simulink model "JingChuJointR"  (R2025b)
settings: Solver=VariableStepAuto  StartTime=0.0  StopTime=10.0  RelTol=1e-3
undefined symbols (not defined in the file or in its folder): X, Y, Z
libraries: sm_lib x486, nesl_utility x6
(part 9 of 9)

== system JingChuJointR/waist_roll1 ==
  Inertia : sm_lib/Body Elements/Inertia  InertiaType=Custom  Mass=1.815  MassUnits=kg  CenterOfMass=[0, 0, 0]  CenterOfMassUnits=m  MomentsOfInertia=[0.002180655, 0.00238951, 0.002296057]  MomentsOfInertiaUnits=kg*m^2  ProductsOfInertia=[-3.6e-08, -8.354199999999999e-05, -8e-09]  ProductsOfInertiaUnits=kg*m^2  GraphicType=None  MarkerShape=Inertia  MarkerSize=20  GraphicVisPropType=SimpleVisualProperties  GraphicDiffuseColor=[0.5 0.5 0.5]  GraphicOpacity=1  GraphicSpecularColor=[0.5 0.5 0.5 1.0]  GraphicAmbientColor=[0.15 0.15 0.15 1.0]  GraphicEmissiveColor=[0.0 0.0 0.0 1.0]  GraphicShininess=75
  InertiaOriginTransform : sm_lib/Frames and Transforms/Rigid Transform  RotationMethod=RotationSequence  FollAlignAxisA=+X  BaseAlignAxisA=+Y  FollAlignAxisB=+Y  BaseAlignAxisB=+Z  RotationStandardAxis=+Z  RotationAngle=0  RotationAngleUnits=deg  RotationArbitraryAxis=[0 0 1]  RotationSequenceAxes=BaseAxes  RotationSequence=XYZ  RotationSequenceAngles=[0, 0, 0]  RotationSequenceAnglesUnits=rad  RotationMatrix=[1 0 0;0 1 0;0 0 1]  Quaternion=[1 0 0 0]  TranslationMethod=Cartesian  TranslationCartesianOffset=[-0.004186, 0, -0.006951]  TranslationCartesianOffsetUnits=m  TranslationStandardAxis=+Z  TranslationStandardOffset=0  TranslationStandardOffsetUnits=m  TranslationROffset=0  TranslationROffsetUnits=m  TranslationThetaOffset=0  TranslationThetaOffsetUnits=deg  TranslationZOffset=0  TranslationZOffsetUnits=m
  ReferenceFrame : sm_lib/Frames and Transforms/Reference Frame
  Visual : sm_lib/Body Elements/File Solid  ExtGeomFileName=./meshes/waist_roll.STL  UnitType=Custom  ExtGeomFileUnits=m  StepReaderType=HEX  ExportConvexHullGeometry=off  InertiaType=Custom  BasedOnType=DensityFromFile  Density=1000  DensityUnits=kg/m^3  Mass=0  MassUnits=kg  CenterOfMass=[0, 0, 0]  CenterOfMassUnits=m  MomentsOfInertia=[0, 0, 0]  MomentsOfInertiaUnits=kg*m^2  ProductsOfInertia=[0, 0, 0]  ProductsOfInertiaUnits=kg*m^2  GraphicType=FromGeometry  MarkerShape=Sphere  MarkerSize=10  GraphicVisPropType=SimpleVisualProperties  GraphicDiffuseColor=[1, 1, 1]  GraphicOpacity=1  GraphicSpecularColor=[0.5 0.5 0.5 1.0]  GraphicAmbientColor=[0.15 0.15 0.15 1.0]  GraphicEmissiveColor=[0.0 0.0 0.0 1.0]  GraphicShininess=75  DoExposeReferenceFrame=on  SerializedFrames=<Frames/>
  VisualOriginTransform : sm_lib/Frames and Transforms/Rigid Transform  RotationMethod=RotationSequence  FollAlignAxisA=+X  BaseAlignAxisA=+Y  FollAlignAxisB=+Y  BaseAlignAxisB=+Z  RotationStandardAxis=+Z  RotationAngle=0  RotationAngleUnits=deg  RotationArbitraryAxis=[0 0 1]  RotationSequenceAxes=BaseAxes  RotationSequence=XYZ  RotationSequenceAngles=[0, 0, 0]  RotationSequenceAnglesUnits=rad  RotationMatrix=[1 0 0;0 1 0;0 0 1]  Quaternion=[1 0 0 0]  TranslationMethod=Cartesian  TranslationCartesianOffset=[0, 0, 0]  TranslationCartesianOffsetUnits=m  TranslationStandardAxis=+Z  TranslationStandardOffset=0  TranslationStandardOffsetUnits=m  TranslationROffset=0  TranslationROffsetUnits=m  TranslationThetaOffset=0  TranslationThetaOffsetUnits=deg  TranslationZOffset=0  TranslationZOffsetUnits=m
  waist_roll_AxisInvTransform : sm_lib/Frames and Transforms/Rigid Transform  RotationMethod=ArbitraryAxis  FollAlignAxisA=+X  BaseAlignAxisA=+Y  FollAlignAxisB=+Y  BaseAlignAxisB=+Z  RotationStandardAxis=+Z  RotationAngle=1.570796326794897  RotationAngleUnits=rad  RotationArbitraryAxis=[-0, 1, 0]  RotationSequenceAxes=FollowerAxes  RotationSequence=XYX  RotationSequenceAngles=[0 0 0]  RotationSequenceAnglesUnits=deg  RotationMatrix=[1 0 0;0 1 0;0 0 1]  Quaternion=[1 0 0 0]  TranslationMethod=Cartesian  TranslationCartesianOffset=[0, 0, 0]  TranslationCartesianOffsetUnits=m  TranslationStandardAxis=+Z  TranslationStandardOffset=0  TranslationStandardOffsetUnits=m  TranslationROffset=0  TranslationROffsetUnits=m  TranslationThetaOffset=0  TranslationThetaOffsetUnits=deg  TranslationZOffset=0  TranslationZOffsetUnits=m
  waist_yaw_AxisTransform : sm_lib/Frames and Transforms/Rigid Transform  RotationMethod=ArbitraryAxis  FollAlignAxisA=+X  BaseAlignAxisA=+Y  FollAlignAxisB=+Y  BaseAlignAxisB=+Z  RotationStandardAxis=+Z  RotationAngle=0  RotationAngleUnits=rad  RotationArbitraryAxis=[1, 0, 0]  RotationSequenceAxes=FollowerAxes  RotationSequence=XYX  RotationSequenceAngles=[0 0 0]  RotationSequenceAnglesUnits=deg  RotationMatrix=[1 0 0;0 1 0;0 0 1]  Quaternion=[1 0 0 0]  TranslationMethod=Cartesian  TranslationCartesianOffset=[0, 0, 0]  TranslationCartesianOffsetUnits=m  TranslationStandardAxis=+Z  TranslationStandardOffset=0  TranslationStandardOffsetUnits=m  TranslationROffset=0  TranslationROffsetUnits=m  TranslationThetaOffset=0  TranslationThetaOffsetUnits=deg  TranslationZOffset=0  TranslationZOffsetUnits=m
  waist_yaw_OriginTransform : sm_lib/Frames and Transforms/Rigid Transform  RotationMethod=RotationSequence  FollAlignAxisA=+X  BaseAlignAxisA=+Y  FollAlignAxisB=+Y  BaseAlignAxisB=+Z  RotationStandardAxis=+Z  RotationAngle=0  RotationAngleUnits=deg  RotationArbitraryAxis=[0 0 1]  RotationSequenceAxes=BaseAxes  RotationSequence=XYZ  RotationSequenceAngles=[0, 0, 0]  RotationSequenceAnglesUnits=rad  RotationMatrix=[1 0 0;0 1 0;0 0 1]  Quaternion=[1 0 0 0]  TranslationMethod=Cartesian  TranslationCartesianOffset=[0, 0, 0]  TranslationCartesianOffsetUnits=m  TranslationStandardAxis=+Z  TranslationStandardOffset=0  TranslationStandardOffsetUnits=m  TranslationROffset=0  TranslationROffsetUnits=m  TranslationThetaOffset=0  TranslationThetaOffsetUnits=deg  TranslationZOffset=0  TranslationZOffsetUnits=m
  F : PMIOPort  Side=Left
  F1 : PMIOPort  Port=2  Side=Right
  connections:
  Inertia/RConn1 -- InertiaOriginTransform/RConn1
  ReferenceFrame/RConn1 -- InertiaOriginTransform/LConn1 -- VisualOriginTransform/LConn1 -- waist_roll_AxisInvTransform/LConn1 -- waist_yaw_OriginTransform/LConn1
  Visual/RConn1 -- VisualOriginTransform/RConn1
  waist_roll_AxisInvTransform/RConn1 -- F/RConn1
  waist_yaw_AxisTransform/RConn1 -- F1/RConn1
  waist_yaw_AxisTransform/LConn1 -- waist_yaw_OriginTransform/RConn1

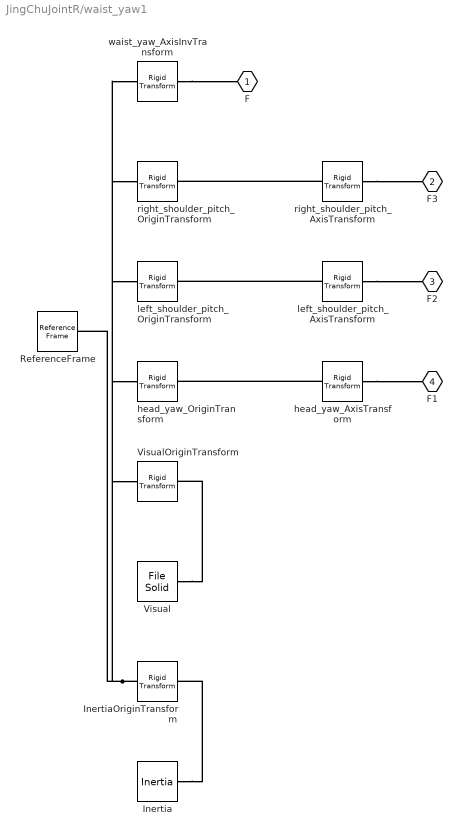
== system JingChuJointR/waist_yaw1 ==
  Inertia : sm_lib/Body Elements/Inertia  InertiaType=Custom  Mass=16.823  MassUnits=kg  CenterOfMass=[0, 0, 0]  CenterOfMassUnits=m  MomentsOfInertia=[0.256789087, 0.21861739, 0.122453074]  MomentsOfInertiaUnits=kg*m^2  ProductsOfInertia=[-0.000143525, 0.007865723, -9.021000000000001e-06]  ProductsOfInertiaUnits=kg*m^2  GraphicType=None  MarkerShape=Inertia  MarkerSize=20  GraphicVisPropType=SimpleVisualProperties  GraphicDiffuseColor=[0.5 0.5 0.5]  GraphicOpacity=1  GraphicSpecularColor=[0.5 0.5 0.5 1.0]  GraphicAmbientColor=[0.15 0.15 0.15 1.0]  GraphicEmissiveColor=[0.0 0.0 0.0 1.0]  GraphicShininess=75
  InertiaOriginTransform : sm_lib/Frames and Transforms/Rigid Transform  RotationMethod=RotationSequence  FollAlignAxisA=+X  BaseAlignAxisA=+Y  FollAlignAxisB=+Y  BaseAlignAxisB=+Z  RotationStandardAxis=+Z  RotationAngle=0  RotationAngleUnits=deg  RotationArbitraryAxis=[0 0 1]  RotationSequenceAxes=BaseAxes  RotationSequence=XYZ  RotationSequenceAngles=[0, 0, 0]  RotationSequenceAnglesUnits=rad  RotationMatrix=[1 0 0;0 1 0;0 0 1]  Quaternion=[1 0 0 0]  TranslationMethod=Cartesian  TranslationCartesianOffset=[-0.04269, 3e-05, 0.24319]  TranslationCartesianOffsetUnits=m  TranslationStandardAxis=+Z  TranslationStandardOffset=0  TranslationStandardOffsetUnits=m  TranslationROffset=0  TranslationROffsetUnits=m  TranslationThetaOffset=0  TranslationThetaOffsetUnits=deg  TranslationZOffset=0  TranslationZOffsetUnits=m
  ReferenceFrame : sm_lib/Frames and Transforms/Reference Frame
  Visual : sm_lib/Body Elements/File Solid  ExtGeomFileName=./meshes/waist_yaw.STL  UnitType=Custom  ExtGeomFileUnits=m  StepReaderType=HEX  ExportConvexHullGeometry=off  InertiaType=Custom  BasedOnType=DensityFromFile  Density=1000  DensityUnits=kg/m^3  Mass=0  MassUnits=kg  CenterOfMass=[0, 0, 0]  CenterOfMassUnits=m  MomentsOfInertia=[0, 0, 0]  MomentsOfInertiaUnits=kg*m^2  ProductsOfInertia=[0, 0, 0]  ProductsOfInertiaUnits=kg*m^2  GraphicType=FromGeometry  MarkerShape=Sphere  MarkerSize=10  GraphicVisPropType=SimpleVisualProperties  GraphicDiffuseColor=[1, 1, 1]  GraphicOpacity=1  GraphicSpecularColor=[0.5 0.5 0.5 1.0]  GraphicAmbientColor=[0.15 0.15 0.15 1.0]  GraphicEmissiveColor=[0.0 0.0 0.0 1.0]  GraphicShininess=75  DoExposeReferenceFrame=on  SerializedFrames=<Frames/>
  VisualOriginTransform : sm_lib/Frames and Transforms/Rigid Transform  RotationMethod=RotationSequence  FollAlignAxisA=+X  BaseAlignAxisA=+Y  FollAlignAxisB=+Y  BaseAlignAxisB=+Z  RotationStandardAxis=+Z  RotationAngle=0  RotationAngleUnits=deg  RotationArbitraryAxis=[0 0 1]  RotationSequenceAxes=BaseAxes  RotationSequence=XYZ  RotationSequenceAngles=[0, 0, 0]  RotationSequenceAnglesUnits=rad  RotationMatrix=[1 0 0;0 1 0;0 0 1]  Quaternion=[1 0 0 0]  TranslationMethod=Cartesian  TranslationCartesianOffset=[0, 0, 0]  TranslationCartesianOffsetUnits=m  TranslationStandardAxis=+Z  TranslationStandardOffset=0  TranslationStandardOffsetUnits=m  TranslationROffset=0  TranslationROffsetUnits=m  TranslationThetaOffset=0  TranslationThetaOffsetUnits=deg  TranslationZOffset=0  TranslationZOffsetUnits=m
  head_yaw_AxisTransform : sm_lib/Frames and Transforms/Rigid Transform  RotationMethod=ArbitraryAxis  FollAlignAxisA=+X  BaseAlignAxisA=+Y  FollAlignAxisB=+Y  BaseAlignAxisB=+Z  RotationStandardAxis=+Z  RotationAngle=3.141592653589793  RotationAngleUnits=rad  RotationArbitraryAxis=[1, 0, 0]  RotationSequenceAxes=FollowerAxes  RotationSequence=XYX  RotationSequenceAngles=[0 0 0]  RotationSequenceAnglesUnits=deg  RotationMatrix=[1 0 0;0 1 0;0 0 1]  Quaternion=[1 0 0 0]  TranslationMethod=Cartesian  TranslationCartesianOffset=[0, 0, 0]  TranslationCartesianOffsetUnits=m  TranslationStandardAxis=+Z  TranslationStandardOffset=0  TranslationStandardOffsetUnits=m  TranslationROffset=0  TranslationROffsetUnits=m  TranslationThetaOffset=0  TranslationThetaOffsetUnits=deg  TranslationZOffset=0  TranslationZOffsetUnits=m
  head_yaw_OriginTransform : sm_lib/Frames and Transforms/Rigid Transform  RotationMethod=RotationSequence  FollAlignAxisA=+X  BaseAlignAxisA=+Y  FollAlignAxisB=+Y  BaseAlignAxisB=+Z  RotationStandardAxis=+Z  RotationAngle=0  RotationAngleUnits=deg  RotationArbitraryAxis=[0 0 1]  RotationSequenceAxes=BaseAxes  RotationSequence=XYZ  RotationSequenceAngles=[0, 0, 0]  RotationSequenceAnglesUnits=rad  RotationMatrix=[1 0 0;0 1 0;0 0 1]  Quaternion=[1 0 0 0]  TranslationMethod=Cartesian  TranslationCartesianOffset=[-0.020000000000003, 0, 0.483]  TranslationCartesianOffsetUnits=m  TranslationStandardAxis=+Z  TranslationStandardOffset=0  TranslationStandardOffsetUnits=m  TranslationROffset=0  TranslationROffsetUnits=m  TranslationThetaOffset=0  TranslationThetaOffsetUnits=deg  TranslationZOffset=0  TranslationZOffsetUnits=m
  left_shoulder_pitch_AxisTransform : sm_lib/Frames and Transforms/Rigid Transform  RotationMethod=ArbitraryAxis  FollAlignAxisA=+X  BaseAlignAxisA=+Y  FollAlignAxisB=+Y  BaseAlignAxisB=+Z  RotationStandardAxis=+Z  RotationAngle=0  RotationAngleUnits=rad  RotationArbitraryAxis=[1, 0, 0]  RotationSequenceAxes=FollowerAxes  RotationSequence=XYX  RotationSequenceAngles=[0 0 0]  RotationSequenceAnglesUnits=deg  RotationMatrix=[1 0 0;0 1 0;0 0 1]  Quaternion=[1 0 0 0]  TranslationMethod=Cartesian  TranslationCartesianOffset=[0, 0, 0]  TranslationCartesianOffsetUnits=m  TranslationStandardAxis=+Z  TranslationStandardOffset=0  TranslationStandardOffsetUnits=m  TranslationROffset=0  TranslationROffsetUnits=m  TranslationThetaOffset=0  TranslationThetaOffsetUnits=deg  TranslationZOffset=0  TranslationZOffsetUnits=m
  left_shoulder_pitch_OriginTransform : sm_lib/Frames and Transforms/Rigid Transform  RotationMethod=RotationSequence  FollAlignAxisA=+X  BaseAlignAxisA=+Y  FollAlignAxisB=+Y  BaseAlignAxisB=+Z  RotationStandardAxis=+Z  RotationAngle=0  RotationAngleUnits=deg  RotationArbitraryAxis=[0 0 1]  RotationSequenceAxes=BaseAxes  RotationSequence=XYZ  RotationSequenceAngles=[1.5707963267949, 0, 0]  RotationSequenceAnglesUnits=rad  RotationMatrix=[1 0 0;0 1 0;0 0 1]  Quaternion=[1 0 0 0]  TranslationMethod=Cartesian  TranslationCartesianOffset=[-0.0199999999999999, 0.13949999999999, 0.404]  TranslationCartesianOffsetUnits=m  TranslationStandardAxis=+Z  TranslationStandardOffset=0  TranslationStandardOffsetUnits=m  TranslationROffset=0  TranslationROffsetUnits=m  TranslationThetaOffset=0  TranslationThetaOffsetUnits=deg  TranslationZOffset=0  TranslationZOffsetUnits=m
  right_shoulder_pitch_AxisTransform : sm_lib/Frames and Transforms/Rigid Transform  RotationMethod=ArbitraryAxis  FollAlignAxisA=+X  BaseAlignAxisA=+Y  FollAlignAxisB=+Y  BaseAlignAxisB=+Z  RotationStandardAxis=+Z  RotationAngle=0  RotationAngleUnits=rad  RotationArbitraryAxis=[1, 0, 0]  RotationSequenceAxes=FollowerAxes  RotationSequence=XYX  RotationSequenceAngles=[0 0 0]  RotationSequenceAnglesUnits=deg  RotationMatrix=[1 0 0;0 1 0;0 0 1]  Quaternion=[1 0 0 0]  TranslationMethod=Cartesian  TranslationCartesianOffset=[0, 0, 0]  TranslationCartesianOffsetUnits=m  TranslationStandardAxis=+Z  TranslationStandardOffset=0  TranslationStandardOffsetUnits=m  TranslationROffset=0  TranslationROffsetUnits=m  TranslationThetaOffset=0  TranslationThetaOffsetUnits=deg  TranslationZOffset=0  TranslationZOffsetUnits=m
  right_shoulder_pitch_OriginTransform : sm_lib/Frames and Transforms/Rigid Transform  RotationMethod=RotationSequence  FollAlignAxisA=+X  BaseAlignAxisA=+Y  FollAlignAxisB=+Y  BaseAlignAxisB=+Z  RotationStandardAxis=+Z  RotationAngle=0  RotationAngleUnits=deg  RotationArbitraryAxis=[0 0 1]  RotationSequenceAxes=BaseAxes  RotationSequence=XYZ  RotationSequenceAngles=[1.5707963267949, 0, 0]  RotationSequenceAnglesUnits=rad  RotationMatrix=[1 0 0;0 1 0;0 0 1]  Quaternion=[1 0 0 0]  TranslationMethod=Cartesian  TranslationCartesianOffset=[-0.0199999999999999, -0.13949999999999, 0.404]  TranslationCartesianOffsetUnits=m  TranslationStandardAxis=+Z  TranslationStandardOffset=0  TranslationStandardOffsetUnits=m  TranslationROffset=0  TranslationROffsetUnits=m  TranslationThetaOffset=0  TranslationThetaOffsetUnits=deg  TranslationZOffset=0  TranslationZOffsetUnits=m
  waist_yaw_AxisInvTransform : sm_lib/Frames and Transforms/Rigid Transform  RotationMethod=ArbitraryAxis  FollAlignAxisA=+X  BaseAlignAxisA=+Y  FollAlignAxisB=+Y  BaseAlignAxisB=+Z  RotationStandardAxis=+Z  RotationAngle=0  RotationAngleUnits=rad  RotationArbitraryAxis=[1, 0, 0]  RotationSequenceAxes=FollowerAxes  RotationSequence=XYX  RotationSequenceAngles=[0 0 0]  RotationSequenceAnglesUnits=deg  RotationMatrix=[1 0 0;0 1 0;0 0 1]  Quaternion=[1 0 0 0]  TranslationMethod=Cartesian  TranslationCartesianOffset=[0, 0, 0]  TranslationCartesianOffsetUnits=m  TranslationStandardAxis=+Z  TranslationStandardOffset=0  TranslationStandardOffsetUnits=m  TranslationROffset=0  TranslationROffsetUnits=m  TranslationThetaOffset=0  TranslationThetaOffsetUnits=deg  TranslationZOffset=0  TranslationZOffsetUnits=m
  F : PMIOPort  Side=Left
  F3 : PMIOPort  Port=2  Side=Right
  F2 : PMIOPort  Port=3  Side=Right
  F1 : PMIOPort  Port=4  Side=Right
  connections:
  Inertia/RConn1 -- InertiaOriginTransform/RConn1
  ReferenceFrame/RConn1 -- InertiaOriginTransform/LConn1 -- VisualOriginTransform/LConn1 -- head_yaw_OriginTransform/LConn1 -- left_shoulder_pitch_OriginTransform/LConn1 -- right_shoulder_pitch_OriginTransform/LConn1 -- waist_yaw_AxisInvTransform/LConn1
  Visual/RConn1 -- VisualOriginTransform/RConn1
  head_yaw_AxisTransform/RConn1 -- F1/RConn1
  head_yaw_AxisTransform/LConn1 -- head_yaw_OriginTransform/RConn1
  left_shoulder_pitch_AxisTransform/RConn1 -- F2/RConn1
  left_shoulder_pitch_AxisTransform/LConn1 -- left_shoulder_pitch_OriginTransform/RConn1
  right_shoulder_pitch_AxisTransform/RConn1 -- F3/RConn1
  right_shoulder_pitch_AxisTransform/LConn1 -- right_shoulder_pitch_OriginTransform/RConn1
  waist_yaw_AxisInvTransform/RConn1 -- F/RConn1

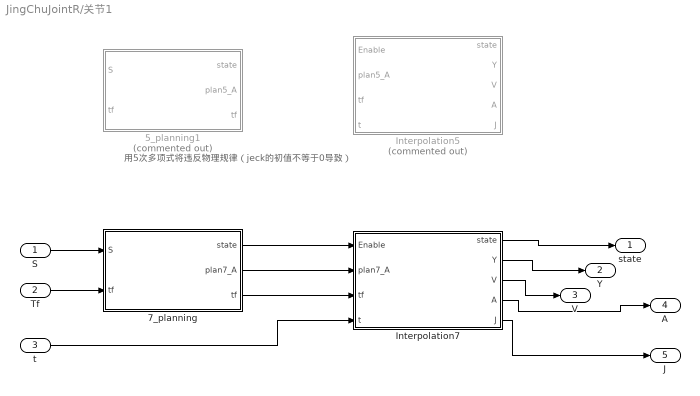
== system JingChuJointR/关节1 ==
  note: 用5次多项式将违反物理规律（jeck的初值不等于0导致）
  S : Inport
  Tf : Inport  Port=2
  t : Inport  Port=3
  5_planning1 : MATLAB Function  Commented=on  TreatAsAtomicUnit=on  mask{g_vs=0, g_ve=0, g_as=0, g_ae=0}
      mask prompts: g_vs "初始速度"; g_ve "末速度"; g_as "初始加速度"; g_ae "末加速度"
  7_planning : MATLAB Function  TreatAsAtomicUnit=on  mask{gv=[0 0], ga=[0 0], gj=[0 0]}
      mask prompts: gv "初末速度"; ga "初末加速度"; gj "初末跃动度"
  Interpolation5 : MATLAB Function  Commented=on  TreatAsAtomicUnit=on
  Interpolation7 : MATLAB Function  TreatAsAtomicUnit=on
  state : Outport
  Y : Outport  Port=2
  V : Outport  Port=3
  A : Outport  Port=4
  J : Outport  Port=5
  wires:
  Interpolation7/1(state) -> state/1
  Interpolation7/2(Y) -> Y/1
  Tf/1 -> 7_planning/2("tf ")
  S/1 -> 7_planning/1(S)
  t/1 -> Interpolation7/4(t)
  Interpolation7/3(V) -> V/1
  Interpolation7/4(A) -> A/1
  Interpolation7/5(J) -> J/1
  7_planning/1(state) -> Interpolation7/1(Enable)
  7_planning/2(plan7_A) -> Interpolation7/2(plan7_A)
  7_planning/3(tf) -> Interpolation7/3(tf)

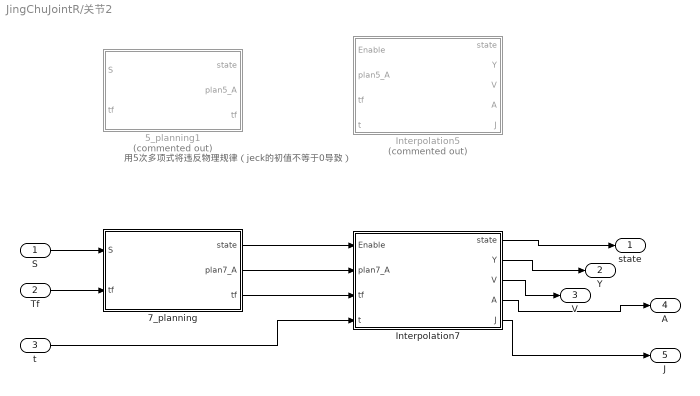
== system JingChuJointR/关节2 ==
  note: 用5次多项式将违反物理规律（jeck的初值不等于0导致）
  S : Inport
  Tf : Inport  Port=2
  t : Inport  Port=3
  5_planning1 : MATLAB Function  Commented=on  TreatAsAtomicUnit=on  mask{g_vs=0, g_ve=0, g_as=0, g_ae=0}
      mask prompts: g_vs "初始速度"; g_ve "末速度"; g_as "初始加速度"; g_ae "末加速度"
  7_planning : MATLAB Function  TreatAsAtomicUnit=on  mask{gv=[0 0], ga=[0 0], gj=[0 0]}
      mask prompts: gv "初末速度"; ga "初末加速度"; gj "初末跃动度"
  Interpolation5 : MATLAB Function  Commented=on  TreatAsAtomicUnit=on
  Interpolation7 : MATLAB Function  TreatAsAtomicUnit=on
  state : Outport
  Y : Outport  Port=2
  V : Outport  Port=3
  A : Outport  Port=4
  J : Outport  Port=5
  wires:
  Interpolation7/1(state) -> state/1
  Interpolation7/2(Y) -> Y/1
  Tf/1 -> 7_planning/2("tf ")
  S/1 -> 7_planning/1(S)
  t/1 -> Interpolation7/4(t)
  Interpolation7/3(V) -> V/1
  Interpolation7/4(A) -> A/1
  Interpolation7/5(J) -> J/1
  7_planning/1(state) -> Interpolation7/1(Enable)
  7_planning/2(plan7_A) -> Interpolation7/2(plan7_A)
  7_planning/3(tf) -> Interpolation7/3(tf)

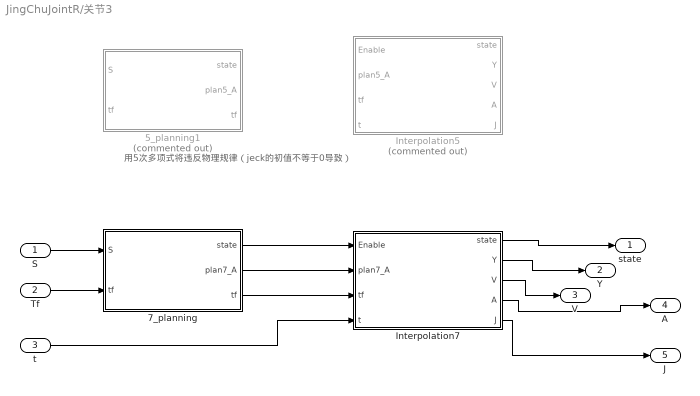
== system JingChuJointR/关节3 ==
  note: 用5次多项式将违反物理规律（jeck的初值不等于0导致）
  S : Inport
  Tf : Inport  Port=2
  t : Inport  Port=3
  5_planning1 : MATLAB Function  Commented=on  TreatAsAtomicUnit=on  mask{g_vs=0, g_ve=0, g_as=0, g_ae=0}
      mask prompts: g_vs "初始速度"; g_ve "末速度"; g_as "初始加速度"; g_ae "末加速度"
  7_planning : MATLAB Function  TreatAsAtomicUnit=on  mask{gv=[0 0], ga=[0 0], gj=[0 0]}
      mask prompts: gv "初末速度"; ga "初末加速度"; gj "初末跃动度"
  Interpolation5 : MATLAB Function  Commented=on  TreatAsAtomicUnit=on
  Interpolation7 : MATLAB Function  TreatAsAtomicUnit=on
  state : Outport
  Y : Outport  Port=2
  V : Outport  Port=3
  A : Outport  Port=4
  J : Outport  Port=5
  wires:
  Interpolation7/1(state) -> state/1
  Interpolation7/2(Y) -> Y/1
  Tf/1 -> 7_planning/2("tf ")
  S/1 -> 7_planning/1(S)
  t/1 -> Interpolation7/4(t)
  Interpolation7/3(V) -> V/1
  Interpolation7/4(A) -> A/1
  Interpolation7/5(J) -> J/1
  7_planning/1(state) -> Interpolation7/1(Enable)
  7_planning/2(plan7_A) -> Interpolation7/2(plan7_A)
  7_planning/3(tf) -> Interpolation7/3(tf)

== system JingChuJointR/Start1/Time ==
  Enable : EnablePort
  Constant : Constant  SampleTime=-1
  Integrator : Integrator
  t : Outport
  wires:
  Constant/1 -> Integrator/1
  Integrator/1 -> t/1

== system JingChuJointR/Start2/Time ==
  Enable : EnablePort
  Constant : Constant  SampleTime=-1
  Integrator : Integrator
  t : Outport
  wires:
  Constant/1 -> Integrator/1
  Integrator/1 -> t/1

== system JingChuJointR/Start3/Time ==
  Enable : EnablePort
  Constant : Constant  SampleTime=-1
  Integrator : Integrator
  t : Outport
  wires:
  Constant/1 -> Integrator/1
  Integrator/1 -> t/1

== matlab function JingChuJointR/关节3/5_planning1 ==
  data: S input; tf input; state output; plan5_A output; g_vs parameter; g_ve parameter; tf output; g_as parameter; g_ae parameter
function [state, plan5_A,tf] =planning5( S,tf,g_vs, g_ve, g_as, g_ae)
% 五次多项式算法主程序
% vs初始速度m/min,ve末速度m/min
% as初始加速度，ae末加速度
% S总位移m,tf为规划时间
% 基础插补规划函数
% 五次多项式速度规划
    a0 = 0 ;
    a1 = g_vs ;
    a2 = g_as/2;
    a3 = (20*S - (8*g_ve + 12 * g_vs )*tf - (3*g_as - g_ae)*tf^2)/(2*tf^3);
    a4 = (-30*S + (14*g_ve + 16 * g_vs )*tf + (3*g_as - 2*g_ae)*tf^2)/(2*tf^4);
    a5 = (12*S - 6*(g_ve + g_vs )*tf + (g_ae - g_as)*tf^2)/(2*tf^5);
  
    state = 1;
    plan5_A = [a0 a1 a2 a3 a4 a5];
    tf =tf ;

end

== matlab function JingChuJointR/关节3/7_planning ==
  data: S input; tf input; state output; plan7_A output; gv parameter; ga parameter; tf output; gj parameter
function [state, plan7_A,tf] =planning7( S,tf,gv,ga,gj)
% 7次多项式算法主程序
% vs初始速度m/min,ve末速度m/min
% as初始加速度，ae末加速度
% S总位移m,tf为规划时间
% 基础插补规划函数
% 五次多项式速度规划

 g_vs = gv(1);
 g_ve = gv(2);
 
 g_as = ga(1);
 g_ae = ga(2);

 g_js = gj(1);
 g_je = gj(2);

    a0 = 0 ;
    a1 = g_vs ;
    a2 = g_as/2;
    a3 = g_js/6;
    a4 = (210*S-tf*((30*g_as-15*g_ae)*tf + (4*g_js+g_je)*tf^2 + 120*g_vs + 90*g_ve)) / (6*tf^4);
    a5 = (-168*S + tf*((20*g_as-14*g_ae)*tf + (2*g_js+g_je)*tf^2 + 90*g_vs +78*g_ve)) / (2*tf^5);
    a6 = (420*S-tf*((45*g_as-39*g_ae)*tf+(4*g_js+3*g_je)*tf^2+216*g_vs+204*g_ve)) / (6*tf^6);
    a7 = (-120*S+tf*((12*g_as-12*g_ae)*tf+(g_js+g_je)*tf*tf+60*g_vs+60*g_ve)) / (6*power(tf,7));
    state = 1;
    plan7_A = [a0 a1 a2 a3 a4 a5 a6 a7];
    tf =tf ;

end

== matlab function JingChuJointR/关节3/Interpolation5 ==
  data: state output; Enable input; Y output; plan5_A input; tf input; t input; V output; A output; J output
function [state, Y,V,A,J]  = Interpolate5(Enable,plan5_A,tf,t)
%% input
a0 = plan5_A(1);
a1 = plan5_A(2);
a2 = plan5_A(3);
a3 = plan5_A(4);
a4 = plan5_A(5);
a5 = plan5_A(6);
Y = 0;
V = 0;
A = 0;
J = 0;
%% output
if Enable == 1
    if t <=tf
    Y = a0 + a1*t + a2*t^2 + a3*t^3 + a4*t^4 + a5*t^5; 
    V = a1 + 2*a2*t + 3*a3*t^2 + 4*a4*t^3 + 5*a5*t^4;
    A = 2*a2 + 6*a3*t + 12*a4*t^2 + 20*a5*t^3;
    J = 6*a3 + 24*a4*t + 60*a5*t^2;
    state =1;
    else
    Y = a0 + a1*tf + a2*tf^2 + a3*tf^3 + a4*tf^4 + a5*tf^5;
    V = a1 + 2*a2*tf + 3*a3*tf^2 + 4*a4*tf^3 + 5*a5*tf^4;
    A = 2*a2 + 6*a3*tf + 12*a4*tf^2 + 20*a5*tf^3;
    J = 0;     % 不是 6*a3 + 24*a4*tf + 60*a5*tf^2 % 由于五次多项式无法指定J的初末值，请注意J不连续
    state = 1;
    end
else 
    Y = 0;
    state = 0;
end
end

== matlab function JingChuJointR/关节3/Interpolation7 ==
  data: state output; Enable input; Y output; plan7_A input; tf input; t input; V output; A output; J output
function [state, Y,V,A,J]  = Interpolate7(Enable,plan7_A,tf,t)
%% input
a0 = plan7_A(1);
a1 = plan7_A(2);
a2 = plan7_A(3);
a3 = plan7_A(4);
a4 = plan7_A(5);
a5 = plan7_A(6);
a6 = plan7_A(7);
a7 = plan7_A(8);
Y = 0;
V = 0;
A = 0;
J = 0;
t0 = 0;
%% output
if Enable == 1
    if t <=tf
    Y = a0+a1*power(t-t0,1)+a2*power(t-t0,2)+a3*power(t-t0,3)+a4*power(t-t0,4)+a5*power(t-t0,5)+a6*power(t-t0,6)+a7*power(t-t0,7);
    V = a1+2*a2*power(t-t0,1)+3*a3*power(t-t0,2)+4*a4*power(t-t0,3)+5*a5*power(t-t0,4)+6*a6*power(t-t0,5)+7*a7*power(t-t0,6);
    A = 2*a2+2*3*a3*power(t-t0,1)+3*4*a4*power(t-t0,2)+4*5*a5*power(t-t0,3)+5*6*a6*power(t-t0,4)+6*7*a7*power(t-t0,5);
    J = 2*3*a3+2*3*4*a4*power(t-t0,1)+3*4*5*a5*power(t-t0,2)+4*5*6*a6*power(t-t0,3)+5*6*7*a7*power(t-t0,4);
    state =1;
    else
    Y = a0+a1*power(tf-t0,1)+a2*power(tf-t0,2)+a3*power(tf-t0,3)+a4*power(tf-t0,4)+a5*power(tf-t0,5)+a6*power(tf-t0,6)+a7*power(tf-t0,7);
    V = a1+2*a2*power(tf-t0,1)+3*a3*power(tf-t0,2)+4*a4*power(tf-t0,3)+5*a5*power(tf-t0,4)+6*a6*power(tf-t0,5)+7*a7*power(tf-t0,6);
    A = 2*a2+2*3*a3*power(tf-t0,1)+3*4*a4*power(tf-t0,2)+4*5*a5*power(tf-t0,3)+5*6*a6*power(tf-t0,4)+6*7*a7*power(tf-t0,5);
    J = 2*3*a3+2*3*4*a4*power(tf-t0,1)+3*4*5*a5*power(tf-t0,2)+4*5*6*a6*power(tf-t0,3)+5*6*7*a7*power(tf-t0,4);
    state = 1;
    end
else 
    Y = 0;
    state = 0;
end
end

== matlab function JingChuJointR/关节1/Interpolation5 ==
  data: state output; Enable input; Y output; plan5_A input; tf input; t input; V output; A output; J output
function [state, Y,V,A,J]  = Interpolate5(Enable,plan5_A,tf,t)
%% input
a0 = plan5_A(1);
a1 = plan5_A(2);
a2 = plan5_A(3);
a3 = plan5_A(4);
a4 = plan5_A(5);
a5 = plan5_A(6);
Y = 0;
V = 0;
A = 0;
J = 0;
%% output
if Enable == 1
    if t <=tf
    Y = a0 + a1*t + a2*t^2 + a3*t^3 + a4*t^4 + a5*t^5; 
    V = a1 + 2*a2*t + 3*a3*t^2 + 4*a4*t^3 + 5*a5*t^4;
    A = 2*a2 + 6*a3*t + 12*a4*t^2 + 20*a5*t^3;
    J = 6*a3 + 24*a4*t + 60*a5*t^2;
    state =1;
    else
    Y = a0 + a1*tf + a2*tf^2 + a3*tf^3 + a4*tf^4 + a5*tf^5;
    V = a1 + 2*a2*tf + 3*a3*tf^2 + 4*a4*tf^3 + 5*a5*tf^4;
    A = 2*a2 + 6*a3*tf + 12*a4*tf^2 + 20*a5*tf^3;
    J = 0;     % 不是 6*a3 + 24*a4*tf + 60*a5*tf^2 % 由于五次多项式无法指定J的初末值，请注意J不连续
    state = 1;
    end
else 
    Y = 0;
    state = 0;
end
end

== matlab function JingChuJointR/关节1/5_planning1 ==
  data: S input; tf input; state output; plan5_A output; g_vs parameter; g_ve parameter; tf output; g_as parameter; g_ae parameter
function [state, plan5_A,tf] =planning5( S,tf,g_vs, g_ve, g_as, g_ae)
% 五次多项式算法主程序
% vs初始速度m/min,ve末速度m/min
% as初始加速度，ae末加速度
% S总位移m,tf为规划时间
% 基础插补规划函数
% 五次多项式速度规划
    a0 = 0 ;
    a1 = g_vs ;
    a2 = g_as/2;
    a3 = (20*S - (8*g_ve + 12 * g_vs )*tf - (3*g_as - g_ae)*tf^2)/(2*tf^3);
    a4 = (-30*S + (14*g_ve + 16 * g_vs )*tf + (3*g_as - 2*g_ae)*tf^2)/(2*tf^4);
    a5 = (12*S - 6*(g_ve + g_vs )*tf + (g_ae - g_as)*tf^2)/(2*tf^5);
  
    state = 1;
    plan5_A = [a0 a1 a2 a3 a4 a5];
    tf =tf ;

end

== matlab function JingChuJointR/关节1/7_planning ==
  data: S input; tf input; state output; plan7_A output; gv parameter; ga parameter; tf output; gj parameter
function [state, plan7_A,tf] =planning7( S,tf,gv,ga,gj)
% 7次多项式算法主程序
% vs初始速度m/min,ve末速度m/min
% as初始加速度，ae末加速度
% S总位移m,tf为规划时间
% 基础插补规划函数
% 五次多项式速度规划

 g_vs = gv(1);
 g_ve = gv(2);
 
 g_as = ga(1);
 g_ae = ga(2);

 g_js = gj(1);
 g_je = gj(2);

    a0 = 0 ;
    a1 = g_vs ;
    a2 = g_as/2;
    a3 = g_js/6;
    a4 = (210*S-tf*((30*g_as-15*g_ae)*tf + (4*g_js+g_je)*tf^2 + 120*g_vs + 90*g_ve)) / (6*tf^4);
    a5 = (-168*S + tf*((20*g_as-14*g_ae)*tf + (2*g_js+g_je)*tf^2 + 90*g_vs +78*g_ve)) / (2*tf^5);
    a6 = (420*S-tf*((45*g_as-39*g_ae)*tf+(4*g_js+3*g_je)*tf^2+216*g_vs+204*g_ve)) / (6*tf^6);
    a7 = (-120*S+tf*((12*g_as-12*g_ae)*tf+(g_js+g_je)*tf*tf+60*g_vs+60*g_ve)) / (6*power(tf,7));
    state = 1;
    plan7_A = [a0 a1 a2 a3 a4 a5 a6 a7];
    tf =tf ;

end

== matlab function JingChuJointR/关节1/Interpolation7 ==
  data: state output; Enable input; Y output; plan7_A input; tf input; t input; V output; A output; J output
function [state, Y,V,A,J]  = Interpolate7(Enable,plan7_A,tf,t)
%% input
a0 = plan7_A(1);
a1 = plan7_A(2);
a2 = plan7_A(3);
a3 = plan7_A(4);
a4 = plan7_A(5);
a5 = plan7_A(6);
a6 = plan7_A(7);
a7 = plan7_A(8);
Y = 0;
V = 0;
A = 0;
J = 0;
t0 = 0;
%% output
if Enable == 1
    if t <=tf
    Y = a0+a1*power(t-t0,1)+a2*power(t-t0,2)+a3*power(t-t0,3)+a4*power(t-t0,4)+a5*power(t-t0,5)+a6*power(t-t0,6)+a7*power(t-t0,7);
    V = a1+2*a2*power(t-t0,1)+3*a3*power(t-t0,2)+4*a4*power(t-t0,3)+5*a5*power(t-t0,4)+6*a6*power(t-t0,5)+7*a7*power(t-t0,6);
    A = 2*a2+2*3*a3*power(t-t0,1)+3*4*a4*power(t-t0,2)+4*5*a5*power(t-t0,3)+5*6*a6*power(t-t0,4)+6*7*a7*power(t-t0,5);
    J = 2*3*a3+2*3*4*a4*power(t-t0,1)+3*4*5*a5*power(t-t0,2)+4*5*6*a6*power(t-t0,3)+5*6*7*a7*power(t-t0,4);
    state =1;
    else
    Y = a0+a1*power(tf-t0,1)+a2*power(tf-t0,2)+a3*power(tf-t0,3)+a4*power(tf-t0,4)+a5*power(tf-t0,5)+a6*power(tf-t0,6)+a7*power(tf-t0,7);
    V = a1+2*a2*power(tf-t0,1)+3*a3*power(tf-t0,2)+4*a4*power(tf-t0,3)+5*a5*power(tf-t0,4)+6*a6*power(tf-t0,5)+7*a7*power(tf-t0,6);
    A = 2*a2+2*3*a3*power(tf-t0,1)+3*4*a4*power(tf-t0,2)+4*5*a5*power(tf-t0,3)+5*6*a6*power(tf-t0,4)+6*7*a7*power(tf-t0,5);
    J = 2*3*a3+2*3*4*a4*power(tf-t0,1)+3*4*5*a5*power(tf-t0,2)+4*5*6*a6*power(tf-t0,3)+5*6*7*a7*power(tf-t0,4);
    state = 1;
    end
else 
    Y = 0;
    state = 0;
end
end

== matlab function JingChuJointR/关节2/5_planning1 ==
  data: S input; tf input; state output; plan5_A output; g_vs parameter; g_ve parameter; tf output; g_as parameter; g_ae parameter
function [state, plan5_A,tf] =planning5( S,tf,g_vs, g_ve, g_as, g_ae)
% 五次多项式算法主程序
% vs初始速度m/min,ve末速度m/min
% as初始加速度，ae末加速度
% S总位移m,tf为规划时间
% 基础插补规划函数
% 五次多项式速度规划
    a0 = 0 ;
    a1 = g_vs ;
    a2 = g_as/2;
    a3 = (20*S - (8*g_ve + 12 * g_vs )*tf - (3*g_as - g_ae)*tf^2)/(2*tf^3);
    a4 = (-30*S + (14*g_ve + 16 * g_vs )*tf + (3*g_as - 2*g_ae)*tf^2)/(2*tf^4);
    a5 = (12*S - 6*(g_ve + g_vs )*tf + (g_ae - g_as)*tf^2)/(2*tf^5);
  
    state = 1;
    plan5_A = [a0 a1 a2 a3 a4 a5];
    tf =tf ;

end

== matlab function JingChuJointR/关节2/7_planning ==
  data: S input; tf input; state output; plan7_A output; gv parameter; ga parameter; tf output; gj parameter
function [state, plan7_A,tf] =planning7( S,tf,gv,ga,gj)
% 7次多项式算法主程序
% vs初始速度m/min,ve末速度m/min
% as初始加速度，ae末加速度
% S总位移m,tf为规划时间
% 基础插补规划函数
% 五次多项式速度规划

 g_vs = gv(1);
 g_ve = gv(2);
 
 g_as = ga(1);
 g_ae = ga(2);

 g_js = gj(1);
 g_je = gj(2);

    a0 = 0 ;
    a1 = g_vs ;
    a2 = g_as/2;
    a3 = g_js/6;
    a4 = (210*S-tf*((30*g_as-15*g_ae)*tf + (4*g_js+g_je)*tf^2 + 120*g_vs + 90*g_ve)) / (6*tf^4);
    a5 = (-168*S + tf*((20*g_as-14*g_ae)*tf + (2*g_js+g_je)*tf^2 + 90*g_vs +78*g_ve)) / (2*tf^5);
    a6 = (420*S-tf*((45*g_as-39*g_ae)*tf+(4*g_js+3*g_je)*tf^2+216*g_vs+204*g_ve)) / (6*tf^6);
    a7 = (-120*S+tf*((12*g_as-12*g_ae)*tf+(g_js+g_je)*tf*tf+60*g_vs+60*g_ve)) / (6*power(tf,7));
    state = 1;
    plan7_A = [a0 a1 a2 a3 a4 a5 a6 a7];
    tf =tf ;

end

== matlab function JingChuJointR/关节2/Interpolation5 ==
  data: state output; Enable input; Y output; plan5_A input; tf input; t input; V output; A output; J output
function [state, Y,V,A,J]  = Interpolate5(Enable,plan5_A,tf,t)
%% input
a0 = plan5_A(1);
a1 = plan5_A(2);
a2 = plan5_A(3);
a3 = plan5_A(4);
a4 = plan5_A(5);
a5 = plan5_A(6);
Y = 0;
V = 0;
A = 0;
J = 0;
%% output
if Enable == 1
    if t <=tf
    Y = a0 + a1*t + a2*t^2 + a3*t^3 + a4*t^4 + a5*t^5; 
    V = a1 + 2*a2*t + 3*a3*t^2 + 4*a4*t^3 + 5*a5*t^4;
    A = 2*a2 + 6*a3*t + 12*a4*t^2 + 20*a5*t^3;
    J = 6*a3 + 24*a4*t + 60*a5*t^2;
    state =1;
    else
    Y = a0 + a1*tf + a2*tf^2 + a3*tf^3 + a4*tf^4 + a5*tf^5;
    V = a1 + 2*a2*tf + 3*a3*tf^2 + 4*a4*tf^3 + 5*a5*tf^4;
    A = 2*a2 + 6*a3*tf + 12*a4*tf^2 + 20*a5*tf^3;
    J = 0;     % 不是 6*a3 + 24*a4*tf + 60*a5*tf^2 % 由于五次多项式无法指定J的初末值，请注意J不连续
    state = 1;
    end
else 
    Y = 0;
    state = 0;
end
end

== matlab function JingChuJointR/关节2/Interpolation7 ==
  data: state output; Enable input; Y output; plan7_A input; tf input; t input; V output; A output; J output
function [state, Y,V,A,J]  = Interpolate7(Enable,plan7_A,tf,t)
%% input
a0 = plan7_A(1);
a1 = plan7_A(2);
a2 = plan7_A(3);
a3 = plan7_A(4);
a4 = plan7_A(5);
a5 = plan7_A(6);
a6 = plan7_A(7);
a7 = plan7_A(8);
Y = 0;
V = 0;
A = 0;
J = 0;
t0 = 0;
%% output
if Enable == 1
    if t <=tf
    Y = a0+a1*power(t-t0,1)+a2*power(t-t0,2)+a3*power(t-t0,3)+a4*power(t-t0,4)+a5*power(t-t0,5)+a6*power(t-t0,6)+a7*power(t-t0,7);
    V = a1+2*a2*power(t-t0,1)+3*a3*power(t-t0,2)+4*a4*power(t-t0,3)+5*a5*power(t-t0,4)+6*a6*power(t-t0,5)+7*a7*power(t-t0,6);
    A = 2*a2+2*3*a3*power(t-t0,1)+3*4*a4*power(t-t0,2)+4*5*a5*power(t-t0,3)+5*6*a6*power(t-t0,4)+6*7*a7*power(t-t0,5);
    J = 2*3*a3+2*3*4*a4*power(t-t0,1)+3*4*5*a5*power(t-t0,2)+4*5*6*a6*power(t-t0,3)+5*6*7*a7*power(t-t0,4);
    state =1;
    else
    Y = a0+a1*power(tf-t0,1)+a2*power(tf-t0,2)+a3*power(tf-t0,3)+a4*power(tf-t0,4)+a5*power(tf-t0,5)+a6*power(tf-t0,6)+a7*power(tf-t0,7);
    V = a1+2*a2*power(tf-t0,1)+3*a3*power(tf-t0,2)+4*a4*power(tf-t0,3)+5*a5*power(tf-t0,4)+6*a6*power(tf-t0,5)+7*a7*power(tf-t0,6);
    A = 2*a2+2*3*a3*power(tf-t0,1)+3*4*a4*power(tf-t0,2)+4*5*a5*power(tf-t0,3)+5*6*a6*power(tf-t0,4)+6*7*a7*power(tf-t0,5);
    J = 2*3*a3+2*3*4*a4*power(tf-t0,1)+3*4*5*a5*power(tf-t0,2)+4*5*6*a6*power(tf-t0,3)+5*6*7*a7*power(tf-t0,4);
    state = 1;
    end
else 
    Y = 0;
    state = 0;
end
end
